simulink model "eg4"  (R2015a)
settings: Solver=ode45  StartTime=0.0  StopTime=10.0  RelTol=1e-3
settings Model: Creator=Ayush Kumar Shah  LastModifiedBy=ayush

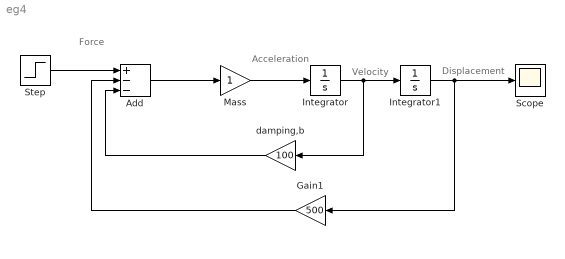
== system eg4 ==
  note: Force
  note: Displacement
  note: Velocity
  note: Acceleration
  Add : Sum  Inputs=+--
  Gain1 : Gain  Gain=500
  Integrator : Integrator
  Integrator1 : Integrator
  "Mass " : Gain
  Scope : Scope
  Step : Step  Time=0  SampleTime=0
  damping,b : Gain  Gain=100
  wires:
  Add/1 -> "Mass "/1
  "Mass "/1 -> Integrator/1
  Integrator/1 -> damping,b/1, Integrator1/1
  Integrator1/1 -> Gain1/1, Scope/1
  damping,b/1 -> Add/3
  Gain1/1 -> Add/2
  Step/1 -> Add/1
